simulink model "Sistema_Teste_Hugo_1"  (R2019a)
settings: Solver=ode23t  StartTime=0.0  StopTime=86400  MaxStep=6  RelTol=1e-3  EnableMultiTasking=on
InitFcn:
  | Dados_do_Sistema
undefined symbols (not defined in the file or in its folder): D1, Dados, Delta
libraries: powerlib x263, powerlib_meascontrol x79, dspsrcs4 x50
(part 3 of 5)

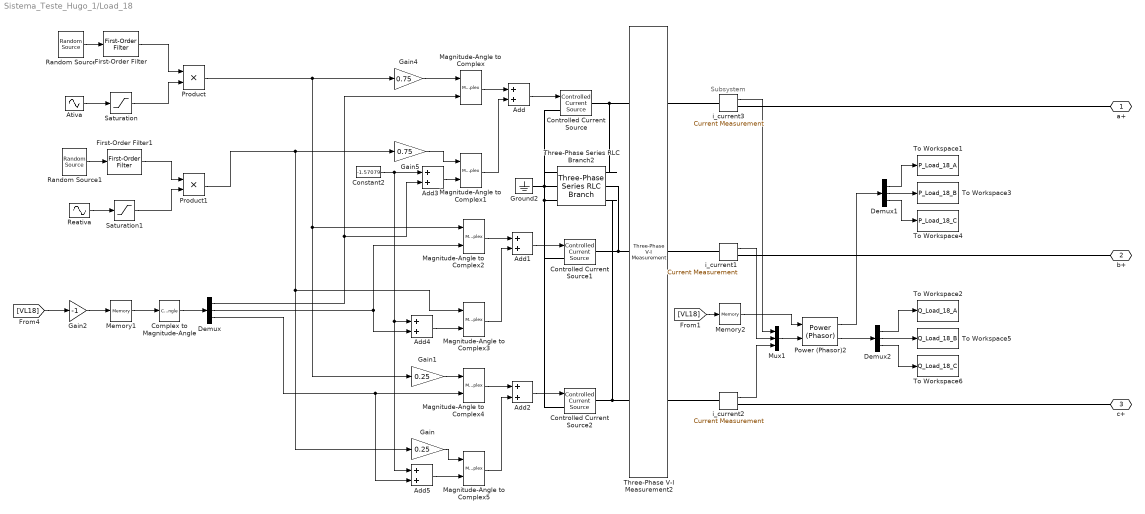
== system Sistema_Teste_Hugo_1/Load_18 ==
  note: Subsystem
  Add{,1..5} (6 alike) : Sum
  Ativa : Sin  Amplitude=21  Frequency=6.9e-5  Phase=-3.14  SampleTime=0
  Complex to Magnitude-Angle : ComplexToMagnitudeAngle  Output=Angle
  Constant2 : Constant  Value=-1.57079
  Controlled Current Source : powerlib/Electrical Sources/Controlled Current Source  Initialize=off  Source_Type=AC  Amplitude=0  Phase=0  Frequency=0  Measurements=None
      settings: SourceProductName=Simscape Electrical
  Controlled Current Source1 : powerlib/Electrical Sources/Controlled Current Source  Initialize=off  Source_Type=AC  Amplitude=0  Phase=0  Frequency=0  Measurements=None
      settings: SourceProductName=Simscape Electrical
  Controlled Current Source2 : powerlib/Electrical Sources/Controlled Current Source  Initialize=off  Source_Type=AC  Amplitude=0  Phase=0  Frequency=0  Measurements=None
      settings: SourceProductName=Simscape Electrical
  Demux : Demux  Outputs=3
  Demux1 : Demux  Outputs=3
  Demux2 : Demux  Outputs=3
  First-Order Filter : powerlib_meascontrol/Filters/First-Order Filter  FilterType=Lowpass  Tc=200  Ts=0  Initialize=on  Vac_Init=[0, 0, 60]  Vdc_Init=1  PlotResponse=off  FreqRange="[0,  200,  1]"
      settings: SourceProductName=Simscape Electrical
  First-Order Filter1 : powerlib_meascontrol/Filters/First-Order Filter  FilterType=Lowpass  Tc=400  Ts=0  Initialize=on  Vac_Init=[0, 0, 60]  Vdc_Init=1  PlotResponse=off  FreqRange="[0,  200,  1]"
      settings: SourceProductName=Simscape Electrical
  Gain : Gain  Gain=0.25
  Gain1 : Gain  Gain=0.25
  Gain2 : Gain  Gain=-1
  Gain4 : Gain  Gain=0.75
  Gain5 : Gain  Gain=0.75
  Ground2 : powerlib/Elements/Ground  LConnTagsString=a
      settings: SourceProductName=Simscape Electrical
  Magnitude-Angle to Complex{,1..5} (6 alike) : MagnitudeAngleToComplex
  Memory1 : Memory
  Memory2 : Memory
  Mux1 : Mux  Inputs=3
  Power (Phasor)2 : powerlib_meascontrol/Measurements/Power (Phasor)
      settings: SourceProductName=Simscape Electrical  SourceProductBaseCode=PS
  Product : Product
  Product1 : Product
  Random Source : dspsrcs4/Random Source  SrcType=Uniform  NormMethod=Ziggurat  CltLength=12  MinVal=0.4  MaxVal=1  MeanVal=0  VarVal=1  RepMode=Repeatable  rawSeed=1  IsInherit=off  SampMode=Discrete  SampTime=200  SampFrame=1  DataType=Single  OutComplex=Real  OutputFrames=on
  Random Source1 : dspsrcs4/Random Source  SrcType=Uniform  NormMethod=Ziggurat  CltLength=12  MinVal=0.75  MaxVal=1.1  MeanVal=0  VarVal=1  RepMode=Repeatable  rawSeed=1  IsInherit=off  SampMode=Discrete  SampTime=400  SampFrame=1  DataType=Single  OutComplex=Real  OutputFrames=on
  Reativa : Sin  Amplitude=9  Frequency=6.9e-5  Phase=-3.14  SampleTime=0
  Saturation : Saturate  UpperLimit=36  LowerLimit=10
  Saturation1 : Saturate  UpperLimit=10  LowerLimit=4
  Three-Phase Series RLC Branch2 : powerlib/Elements/Three-Phase Series RLC Branch  LConnTagsString=A|B|C  RConnTagsString=A|B|C  BranchType=RC  Resistance=0.0001  Inductance=5.46e-6  Capacitance=1e-9  Measurements=None
      settings: SourceProductName=Simscape Electrical
  Three-Phase V-I Measurement2 : powerlib/Measurements/Three-Phase V-I Measurement  VoltageMeasurement=phase-to-ground  SetLabelV=on  LabelV=VL18  Vpu=off  VpuLL=off  CurrentMeasurement=no  SetLabelI=on  LabelI=IL18  Ipu=off  Pbase=100e6  Vbase=500e3  OutputType=Complex  PhasorSimulation=on  PSBequivalent=0
      settings: SourceProductName=Simscape Electrical
  To Workspace1 : ToWorkspace  VariableName=P_Load_18_A  SampleTime=-1
  To Workspace2 : ToWorkspace  VariableName=Q_Load_18_A  SampleTime=-1
  To Workspace3 : ToWorkspace  VariableName=P_Load_18_B  SampleTime=-1
  To Workspace4 : ToWorkspace  VariableName=P_Load_18_C  SampleTime=-1
  To Workspace5 : ToWorkspace  VariableName=Q_Load_18_B  SampleTime=-1
  To Workspace6 : ToWorkspace  VariableName=Q_Load_18_C  SampleTime=-1
  i_current1 : powerlib/Measurements/Current Measurement  PhasorSimulation=on  OutputType=Complex  PSBequivalent=0
      settings: SourceProductName=Simscape Electrical
  i_current2 : powerlib/Measurements/Current Measurement  PhasorSimulation=on  OutputType=Complex  PSBequivalent=0
      settings: SourceProductName=Simscape Electrical
  i_current3 : powerlib/Measurements/Current Measurement  PhasorSimulation=on  OutputType=Complex  PSBequivalent=0
      settings: SourceProductName=Simscape Electrical
  a+ : PMIOPort  Side=Right
  b+ : PMIOPort  Port=2  Side=Right
  c+ : PMIOPort  Port=3  Side=Right
  wires:
  Ativa/1 -> Saturation/1
  Saturation/1 -> Product/2
  Random Source/1 -> First-Order Filter/1
  First-Order Filter/1 -> Product/1
  Reativa/1 -> Saturation1/1
  First-Order Filter1/1 -> Product1/1
  Random Source1/1 -> First-Order Filter1/1
  Saturation1/1 -> Product1/2
  Add/1 -> Controlled Current Source/1
  Magnitude-Angle to Complex/1 -> Add/1
  Magnitude-Angle to Complex1/1 -> Add/2
  Add1/1 -> Controlled Current Source1/1
  Magnitude-Angle to Complex2/1 -> Add1/1
  Magnitude-Angle to Complex3/1 -> Add1/2
  Add2/1 -> Controlled Current Source2/1
  Magnitude-Angle to Complex4/1 -> Add2/1
  Magnitude-Angle to Complex5/1 -> Add2/2
  Complex to Magnitude-Angle/1 -> Demux/1
  Demux/1 -> Magnitude-Angle to Complex/2, Add3/2
  Constant2/1 -> Add5/1, Add4/1, Add3/1
  Add3/1 -> Magnitude-Angle to Complex1/2
  Demux/2 -> Add4/2, Magnitude-Angle to Complex2/2
  Add4/1 -> Magnitude-Angle to Complex3/2
  Demux/3 -> Magnitude-Angle to Complex4/2, Add5/2
  Add5/1 -> Magnitude-Angle to Complex5/2
  [VL18] -> Gain2/1
  Memory1/1 -> Complex to Magnitude-Angle/1
  Product/1 -> Gain4/1, Magnitude-Angle to Complex2/1, Gain1/1
  Product1/1 -> Magnitude-Angle to Complex3/1, Gain/1, Gain5/1
  Gain1/1 -> Magnitude-Angle to Complex4/1
  Gain/1 -> Magnitude-Angle to Complex5/1
  Gain4/1 -> Magnitude-Angle to Complex/1
  Gain5/1 -> Magnitude-Angle to Complex1/1
  Gain2/1 -> Memory1/1
  Demux1/1 -> To Workspace1/1
  i_current3/1 -> Mux1/1
  Demux1/3 -> To Workspace4/1
  Demux2/2 -> To Workspace5/1
  Demux2/3 -> To Workspace6/1
  Memory2/1 -> Power (Phasor)2/1
  Demux1/2 -> To Workspace3/1
  i_current2/1 -> Mux1/3
  i_current1/1 -> Mux1/2
  Demux2/1 -> To Workspace2/1
  Mux1/1 -> Power (Phasor)2/2
  Power (Phasor)2/2 -> Demux2/1
  [VL18] -> Memory2/1
  Power (Phasor)2/1 -> Demux1/1
  connections:
  Controlled Current Source/RConn1 -- Three-Phase Series RLC Branch2/LConn1 -- Three-Phase V-I Measurement2/RConn1
  Controlled Current Source1/RConn1 -- Three-Phase Series RLC Branch2/LConn2 -- Three-Phase V-I Measurement2/RConn2
  Controlled Current Source2/RConn1 -- Three-Phase Series RLC Branch2/LConn3 -- Three-Phase V-I Measurement2/RConn3
  Ground2/LConn1 -- Controlled Current Source1/LConn1 -- Controlled Current Source2/LConn1 -- Three-Phase Series RLC Branch2/RConn3 -- Three-Phase Series RLC Branch2/RConn1 -- Controlled Current Source/LConn1 -- Three-Phase Series RLC Branch2/RConn2
  Three-Phase V-I Measurement2/LConn2 -- i_current1/LConn1
  a+/RConn1 -- i_current3/RConn1
  c+/RConn1 -- i_current2/RConn1
  b+/RConn1 -- i_current1/RConn1
  Three-Phase V-I Measurement2/LConn1 -- i_current3/LConn1
  Three-Phase V-I Measurement2/LConn3 -- i_current2/LConn1

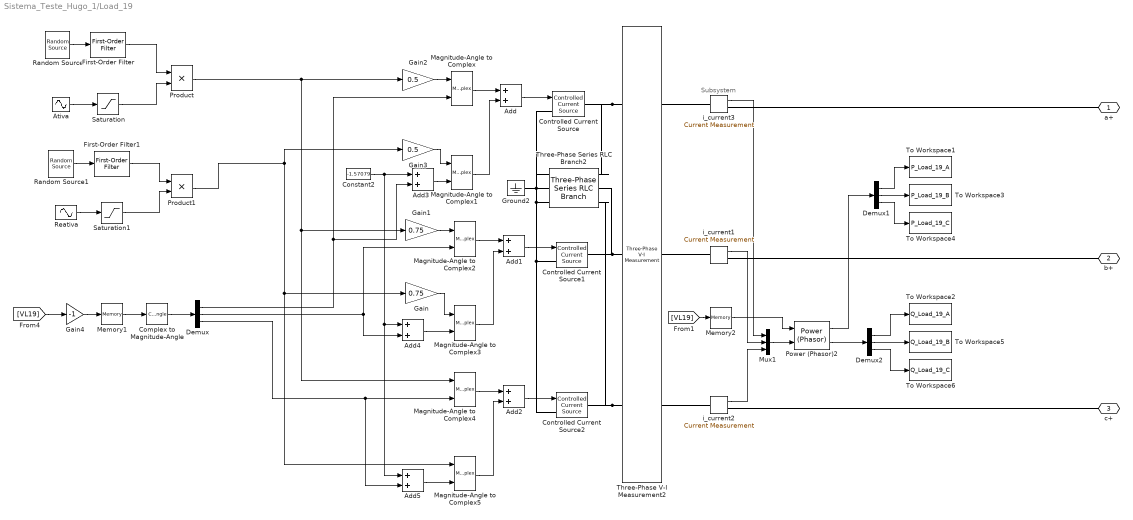
== system Sistema_Teste_Hugo_1/Load_19 ==
  note: Subsystem
  Add{,1..5} (6 alike) : Sum
  Ativa : Sin  Amplitude=22  Frequency=6.9e-5  Phase=-3.14  SampleTime=0
  Complex to Magnitude-Angle : ComplexToMagnitudeAngle  Output=Angle
  Constant2 : Constant  Value=-1.57079
  Controlled Current Source : powerlib/Electrical Sources/Controlled Current Source  Initialize=off  Source_Type=AC  Amplitude=0  Phase=0  Frequency=0  Measurements=None
      settings: SourceProductName=Simscape Electrical
  Controlled Current Source1 : powerlib/Electrical Sources/Controlled Current Source  Initialize=off  Source_Type=AC  Amplitude=0  Phase=0  Frequency=0  Measurements=None
      settings: SourceProductName=Simscape Electrical
  Controlled Current Source2 : powerlib/Electrical Sources/Controlled Current Source  Initialize=off  Source_Type=AC  Amplitude=0  Phase=0  Frequency=0  Measurements=None
      settings: SourceProductName=Simscape Electrical
  Demux : Demux  Outputs=3
  Demux1 : Demux  Outputs=3
  Demux2 : Demux  Outputs=3
  First-Order Filter : powerlib_meascontrol/Filters/First-Order Filter  FilterType=Lowpass  Tc=200  Ts=0  Initialize=on  Vac_Init=[0, 0, 60]  Vdc_Init=1  PlotResponse=off  FreqRange="[0,  200,  1]"
      settings: SourceProductName=Simscape Electrical
  First-Order Filter1 : powerlib_meascontrol/Filters/First-Order Filter  FilterType=Lowpass  Tc=400  Ts=0  Initialize=on  Vac_Init=[0, 0, 60]  Vdc_Init=1  PlotResponse=off  FreqRange="[0,  200,  1]"
      settings: SourceProductName=Simscape Electrical
  Gain : Gain  Gain=0.75
  Gain1 : Gain  Gain=0.75
  Gain2 : Gain  Gain=0.5
  Gain3 : Gain  Gain=0.5
  Gain4 : Gain  Gain=-1
  Ground2 : powerlib/Elements/Ground  LConnTagsString=a
      settings: SourceProductName=Simscape Electrical
  Magnitude-Angle to Complex{,1..5} (6 alike) : MagnitudeAngleToComplex
  Memory1 : Memory
  Memory2 : Memory
  Mux1 : Mux  Inputs=3
  Power (Phasor)2 : powerlib_meascontrol/Measurements/Power (Phasor)
      settings: SourceProductName=Simscape Electrical  SourceProductBaseCode=PS
  Product : Product
  Product1 : Product
  Random Source : dspsrcs4/Random Source  SrcType=Uniform  NormMethod=Ziggurat  CltLength=12  MinVal=0.6  MaxVal=1  MeanVal=0  VarVal=1  RepMode=Repeatable  rawSeed=1  IsInherit=off  SampMode=Discrete  SampTime=200  SampFrame=1  DataType=Single  OutComplex=Real  OutputFrames=on
  Random Source1 : dspsrcs4/Random Source  SrcType=Uniform  NormMethod=Ziggurat  CltLength=12  MinVal=0.8  MaxVal=1  MeanVal=0  VarVal=1  RepMode=Repeatable  rawSeed=1  IsInherit=off  SampMode=Discrete  SampTime=400  SampFrame=1  DataType=Single  OutComplex=Real  OutputFrames=on
  Reativa : Sin  Amplitude=8  Frequency=6.9e-5  Phase=-3.14  SampleTime=0
  Saturation : Saturate  UpperLimit=24  LowerLimit=11
  Saturation1 : Saturate  UpperLimit=9  LowerLimit=7
  Three-Phase Series RLC Branch2 : powerlib/Elements/Three-Phase Series RLC Branch  LConnTagsString=A|B|C  RConnTagsString=A|B|C  BranchType=RC  Resistance=0.0001  Inductance=5.46e-6  Capacitance=1e-9  Measurements=None
      settings: SourceProductName=Simscape Electrical
  Three-Phase V-I Measurement2 : powerlib/Measurements/Three-Phase V-I Measurement  VoltageMeasurement=phase-to-ground  SetLabelV=on  LabelV=VL19  Vpu=off  VpuLL=off  CurrentMeasurement=no  SetLabelI=on  LabelI=IL19  Ipu=off  Pbase=100e6  Vbase=500e3  OutputType=Complex  PhasorSimulation=on  PSBequivalent=0
      settings: SourceProductName=Simscape Electrical
  To Workspace1 : ToWorkspace  VariableName=P_Load_19_A  SampleTime=-1
  To Workspace2 : ToWorkspace  VariableName=Q_Load_19_A  SampleTime=-1
  To Workspace3 : ToWorkspace  VariableName=P_Load_19_B  SampleTime=-1
  To Workspace4 : ToWorkspace  VariableName=P_Load_19_C  SampleTime=-1
  To Workspace5 : ToWorkspace  VariableName=Q_Load_19_B  SampleTime=-1
  To Workspace6 : ToWorkspace  VariableName=Q_Load_19_C  SampleTime=-1
  i_current1 : powerlib/Measurements/Current Measurement  PhasorSimulation=on  OutputType=Complex  PSBequivalent=0
      settings: SourceProductName=Simscape Electrical
  i_current2 : powerlib/Measurements/Current Measurement  PhasorSimulation=on  OutputType=Complex  PSBequivalent=0
      settings: SourceProductName=Simscape Electrical
  i_current3 : powerlib/Measurements/Current Measurement  PhasorSimulation=on  OutputType=Complex  PSBequivalent=0
      settings: SourceProductName=Simscape Electrical
  a+ : PMIOPort  Side=Right
  b+ : PMIOPort  Port=2  Side=Right
  c+ : PMIOPort  Port=3  Side=Right
  wires:
  Ativa/1 -> Saturation/1
  Saturation/1 -> Product/2
  Random Source/1 -> First-Order Filter/1
  First-Order Filter/1 -> Product/1
  Reativa/1 -> Saturation1/1
  First-Order Filter1/1 -> Product1/1
  Random Source1/1 -> First-Order Filter1/1
  Saturation1/1 -> Product1/2
  Add/1 -> Controlled Current Source/1
  Magnitude-Angle to Complex/1 -> Add/1
  Magnitude-Angle to Complex1/1 -> Add/2
  Add1/1 -> Controlled Current Source1/1
  Magnitude-Angle to Complex2/1 -> Add1/1
  Magnitude-Angle to Complex3/1 -> Add1/2
  Add2/1 -> Controlled Current Source2/1
  Magnitude-Angle to Complex4/1 -> Add2/1
  Magnitude-Angle to Complex5/1 -> Add2/2
  Complex to Magnitude-Angle/1 -> Demux/1
  Demux/1 -> Magnitude-Angle to Complex/2, Add3/2
  Constant2/1 -> Add5/1, Add4/1, Add3/1
  Add3/1 -> Magnitude-Angle to Complex1/2
  Demux/2 -> Add4/2, Magnitude-Angle to Complex2/2
  Add4/1 -> Magnitude-Angle to Complex3/2
  Demux/3 -> Magnitude-Angle to Complex4/2, Add5/2
  Add5/1 -> Magnitude-Angle to Complex5/2
  [VL19] -> Gain4/1
  Memory1/1 -> Complex to Magnitude-Angle/1
  Gain1/1 -> Magnitude-Angle to Complex2/1
  Gain/1 -> Magnitude-Angle to Complex3/1
  Product/1 -> Gain2/1, Magnitude-Angle to Complex4/1, Gain1/1
  Product1/1 -> Gain3/1, Magnitude-Angle to Complex5/1, Gain/1
  Gain4/1 -> Memory1/1
  Gain2/1 -> Magnitude-Angle to Complex/1
  Gain3/1 -> Magnitude-Angle to Complex1/1
  Power (Phasor)2/2 -> Demux2/1
  Demux2/1 -> To Workspace2/1
  Power (Phasor)2/1 -> Demux1/1
  i_current3/1 -> Mux1/1
  i_current1/1 -> Mux1/2
  Demux2/3 -> To Workspace6/1
  Demux1/3 -> To Workspace4/1
  Memory2/1 -> Power (Phasor)2/1
  Demux2/2 -> To Workspace5/1
  i_current2/1 -> Mux1/3
  [VL19] -> Memory2/1
  Demux1/1 -> To Workspace1/1
  Demux1/2 -> To Workspace3/1
  Mux1/1 -> Power (Phasor)2/2
  connections:
  Three-Phase V-I Measurement2/RConn1 -- Controlled Current Source/RConn1 -- Three-Phase Series RLC Branch2/LConn1
  Three-Phase V-I Measurement2/RConn2 -- Controlled Current Source1/RConn1 -- Three-Phase Series RLC Branch2/LConn2
  Three-Phase V-I Measurement2/RConn3 -- Controlled Current Source2/RConn1 -- Three-Phase Series RLC Branch2/LConn3
  Controlled Current Source1/LConn1 -- Three-Phase Series RLC Branch2/RConn3 -- Three-Phase Series RLC Branch2/RConn1 -- Controlled Current Source/LConn1 -- Three-Phase Series RLC Branch2/RConn2 -- Ground2/LConn1 -- Controlled Current Source2/LConn1
  b+/RConn1 -- i_current1/RConn1
  c+/RConn1 -- i_current2/RConn1
  Three-Phase V-I Measurement2/LConn2 -- i_current1/LConn1
  a+/RConn1 -- i_current3/RConn1
  Three-Phase V-I Measurement2/LConn3 -- i_current2/LConn1
  Three-Phase V-I Measurement2/LConn1 -- i_current3/LConn1

== system Sistema_Teste_Hugo_1/Load_21 ==
  note: Subsystem
  Add{,1..5} (6 alike) : Sum
  Ativa : Sin  Amplitude=16  Frequency=6.9e-5  Phase=-3.14  SampleTime=0
  Complex to Magnitude-Angle : ComplexToMagnitudeAngle  Output=Angle
  Constant2 : Constant  Value=-1.57079
  Controlled Current Source : powerlib/Electrical Sources/Controlled Current Source  Initialize=off  Source_Type=AC  Amplitude=0  Phase=0  Frequency=0  Measurements=None
      settings: SourceProductName=Simscape Electrical
  Controlled Current Source1 : powerlib/Electrical Sources/Controlled Current Source  Initialize=off  Source_Type=AC  Amplitude=0  Phase=0  Frequency=0  Measurements=None
      settings: SourceProductName=Simscape Electrical
  Controlled Current Source2 : powerlib/Electrical Sources/Controlled Current Source  Initialize=off  Source_Type=AC  Amplitude=0  Phase=0  Frequency=0  Measurements=None
      settings: SourceProductName=Simscape Electrical
  Demux : Demux  Outputs=3
  Demux1 : Demux  Outputs=3
  Demux2 : Demux  Outputs=3
  First-Order Filter : powerlib_meascontrol/Filters/First-Order Filter  FilterType=Lowpass  Tc=200  Ts=0  Initialize=on  Vac_Init=[0, 0, 60]  Vdc_Init=1  PlotResponse=off  FreqRange="[0,  200,  1]"
      settings: SourceProductName=Simscape Electrical
  First-Order Filter1 : powerlib_meascontrol/Filters/First-Order Filter  FilterType=Lowpass  Tc=400  Ts=0  Initialize=on  Vac_Init=[0, 0, 60]  Vdc_Init=1  PlotResponse=off  FreqRange="[0,  200,  1]"
      settings: SourceProductName=Simscape Electrical
  Gain : Gain  Gain=0.25
  Gain1 : Gain  Gain=0.25
  Gain2 : Gain  Gain=0
  Gain3 : Gain  Gain=0
  Gain4 : Gain  Gain=-1
  Ground2 : powerlib/Elements/Ground  LConnTagsString=a
      settings: SourceProductName=Simscape Electrical
  Magnitude-Angle to Complex{,1..5} (6 alike) : MagnitudeAngleToComplex
  Memory1 : Memory
  Memory2 : Memory
  Mux1 : Mux  Inputs=3
  Power (Phasor)2 : powerlib_meascontrol/Measurements/Power (Phasor)
      settings: SourceProductName=Simscape Electrical  SourceProductBaseCode=PS
  Product : Product
  Product1 : Product
  Random Source : dspsrcs4/Random Source  SrcType=Uniform  NormMethod=Ziggurat  CltLength=12  MinVal=0.75  MaxVal=1  MeanVal=0  VarVal=1  RepMode=Repeatable  rawSeed=1  IsInherit=off  SampMode=Discrete  SampTime=200  SampFrame=1  DataType=Single  OutComplex=Real  OutputFrames=on
  Random Source1 : dspsrcs4/Random Source  SrcType=Uniform  NormMethod=Ziggurat  CltLength=12  MinVal=0.8  MaxVal=1  MeanVal=0  VarVal=1  RepMode=Repeatable  rawSeed=1  IsInherit=off  SampMode=Discrete  SampTime=400  SampFrame=1  DataType=Single  OutComplex=Real  OutputFrames=on
  Reativa : Sin  Amplitude=9  Frequency=6.9e-5  Phase=-3.14  SampleTime=0
  Saturation : Saturate  UpperLimit=24  LowerLimit=14
  Saturation1 : Saturate  UpperLimit=12  LowerLimit=8
  Three-Phase Series RLC Branch2 : powerlib/Elements/Three-Phase Series RLC Branch  LConnTagsString=A|B|C  RConnTagsString=A|B|C  BranchType=RC  Resistance=0.0001  Inductance=5.46e-6  Capacitance=1e-9  Measurements=None
      settings: SourceProductName=Simscape Electrical
  Three-Phase V-I Measurement2 : powerlib/Measurements/Three-Phase V-I Measurement  VoltageMeasurement=phase-to-ground  SetLabelV=on  LabelV=VL21  Vpu=off  VpuLL=off  CurrentMeasurement=no  SetLabelI=on  LabelI=IL21  Ipu=off  Pbase=100e6  Vbase=500e3  OutputType=Complex  PhasorSimulation=on  PSBequivalent=0
      settings: SourceProductName=Simscape Electrical
  To Workspace1 : ToWorkspace  VariableName=P_Load_21_A  SampleTime=-1
  To Workspace2 : ToWorkspace  VariableName=Q_Load_21_A  SampleTime=-1
  To Workspace3 : ToWorkspace  VariableName=P_Load_21_B  SampleTime=-1
  To Workspace4 : ToWorkspace  VariableName=P_Load_21_C  SampleTime=-1
  To Workspace5 : ToWorkspace  VariableName=Q_Load_21_B  SampleTime=-1
  To Workspace6 : ToWorkspace  VariableName=Q_Load_21_C  SampleTime=-1
  i_current1 : powerlib/Measurements/Current Measurement  PhasorSimulation=on  OutputType=Complex  PSBequivalent=0
      settings: SourceProductName=Simscape Electrical
  i_current2 : powerlib/Measurements/Current Measurement  PhasorSimulation=on  OutputType=Complex  PSBequivalent=0
      settings: SourceProductName=Simscape Electrical
  i_current3 : powerlib/Measurements/Current Measurement  PhasorSimulation=on  OutputType=Complex  PSBequivalent=0
      settings: SourceProductName=Simscape Electrical
  a+ : PMIOPort  Side=Right
  b+ : PMIOPort  Port=2  Side=Right
  c+ : PMIOPort  Port=3  Side=Right
  wires:
  Ativa/1 -> Saturation/1
  Saturation/1 -> Product/2
  Random Source/1 -> First-Order Filter/1
  First-Order Filter/1 -> Product/1
  Reativa/1 -> Saturation1/1
  First-Order Filter1/1 -> Product1/1
  Random Source1/1 -> First-Order Filter1/1
  Saturation1/1 -> Product1/2
  Add/1 -> Controlled Current Source/1
  Magnitude-Angle to Complex/1 -> Add/1
  Magnitude-Angle to Complex1/1 -> Add/2
  Add1/1 -> Controlled Current Source1/1
  Magnitude-Angle to Complex2/1 -> Add1/1
  Magnitude-Angle to Complex3/1 -> Add1/2
  Add2/1 -> Controlled Current Source2/1
  Magnitude-Angle to Complex4/1 -> Add2/1
  Magnitude-Angle to Complex5/1 -> Add2/2
  Complex to Magnitude-Angle/1 -> Demux/1
  Demux/1 -> Magnitude-Angle to Complex/2, Add3/2
  Constant2/1 -> Add5/1, Add4/1, Add3/1
  Add3/1 -> Magnitude-Angle to Complex1/2
  Demux/2 -> Add4/2, Magnitude-Angle to Complex2/2
  Add4/1 -> Magnitude-Angle to Complex3/2
  Demux/3 -> Magnitude-Angle to Complex4/2, Add5/2
  Add5/1 -> Magnitude-Angle to Complex5/2
  [VL21] -> Gain4/1
  Memory1/1 -> Complex to Magnitude-Angle/1
  Product/1 -> Gain2/1, Magnitude-Angle to Complex2/1, Gain1/1
  Product1/1 -> Gain3/1, Magnitude-Angle to Complex3/1, Gain/1
  Gain4/1 -> Memory1/1
  Gain2/1 -> Magnitude-Angle to Complex/1
  Gain3/1 -> Magnitude-Angle to Complex1/1
  Gain/1 -> Magnitude-Angle to Complex5/1
  Gain1/1 -> Magnitude-Angle to Complex4/1
  Demux2/2 -> To Workspace5/1
  [VL21] -> Memory2/1
  Memory2/1 -> Power (Phasor)2/1
  Demux1/1 -> To Workspace1/1
  i_current2/1 -> Mux1/3
  i_current3/1 -> Mux1/1
  Power (Phasor)2/1 -> Demux1/1
  Demux1/2 -> To Workspace3/1
  i_current1/1 -> Mux1/2
  Demux2/1 -> To Workspace2/1
  Power (Phasor)2/2 -> Demux2/1
  Demux2/3 -> To Workspace6/1
  Mux1/1 -> Power (Phasor)2/2
  Demux1/3 -> To Workspace4/1
  connections:
  Three-Phase V-I Measurement2/RConn1 -- Controlled Current Source/RConn1 -- Three-Phase Series RLC Branch2/LConn1
  Three-Phase V-I Measurement2/RConn2 -- Controlled Current Source1/RConn1 -- Three-Phase Series RLC Branch2/LConn2
  Three-Phase V-I Measurement2/RConn3 -- Controlled Current Source2/RConn1 -- Three-Phase Series RLC Branch2/LConn3
  Controlled Current Source1/LConn1 -- Three-Phase Series RLC Branch2/RConn3 -- Three-Phase Series RLC Branch2/RConn1 -- Controlled Current Source/LConn1 -- Three-Phase Series RLC Branch2/RConn2 -- Ground2/LConn1 -- Controlled Current Source2/LConn1
  a+/RConn1 -- i_current3/RConn1
  b+/RConn1 -- i_current1/RConn1
  Three-Phase V-I Measurement2/LConn2 -- i_current1/LConn1
  Three-Phase V-I Measurement2/LConn3 -- i_current2/LConn1
  c+/RConn1 -- i_current2/RConn1
  Three-Phase V-I Measurement2/LConn1 -- i_current3/LConn1

== system Sistema_Teste_Hugo_1/Load_23 ==
  note: Subsystem
  Add{,1..5} (6 alike) : Sum
  Ativa : Sin  Amplitude=22  Frequency=6.9e-5  Phase=-3.14  SampleTime=0
  Complex to Magnitude-Angle : ComplexToMagnitudeAngle  Output=Angle
  Constant2 : Constant  Value=-1.57079
  Controlled Current Source : powerlib/Electrical Sources/Controlled Current Source  Initialize=off  Source_Type=AC  Amplitude=0  Phase=0  Frequency=0  Measurements=None
      settings: SourceProductName=Simscape Electrical
  Controlled Current Source1 : powerlib/Electrical Sources/Controlled Current Source  Initialize=off  Source_Type=AC  Amplitude=0  Phase=0  Frequency=0  Measurements=None
      settings: SourceProductName=Simscape Electrical
  Controlled Current Source2 : powerlib/Electrical Sources/Controlled Current Source  Initialize=off  Source_Type=AC  Amplitude=0  Phase=0  Frequency=0  Measurements=None
      settings: SourceProductName=Simscape Electrical
  Demux : Demux  Outputs=3
  Demux1 : Demux  Outputs=3
  Demux2 : Demux  Outputs=3
  First-Order Filter : powerlib_meascontrol/Filters/First-Order Filter  FilterType=Lowpass  Tc=200  Ts=0  Initialize=on  Vac_Init=[0, 0, 60]  Vdc_Init=1  PlotResponse=off  FreqRange="[0,  200,  1]"
      settings: SourceProductName=Simscape Electrical
  First-Order Filter1 : powerlib_meascontrol/Filters/First-Order Filter  FilterType=Lowpass  Tc=400  Ts=0  Initialize=on  Vac_Init=[0, 0, 60]  Vdc_Init=1  PlotResponse=off  FreqRange="[0,  200,  1]"
      settings: SourceProductName=Simscape Electrical
  Gain : Gain  Gain=1.25
  Gain1 : Gain  Gain=1.25
  Gain2 : Gain  Gain=2
  Gain3 : Gain  Gain=2
  Gain4 : Gain  Gain=-1
  Ground2 : powerlib/Elements/Ground  LConnTagsString=a
      settings: SourceProductName=Simscape Electrical
  Magnitude-Angle to Complex{,1..5} (6 alike) : MagnitudeAngleToComplex
  Memory1 : Memory
  Memory2 : Memory
  Mux1 : Mux  Inputs=3
  Power (Phasor)2 : powerlib_meascontrol/Measurements/Power (Phasor)
      settings: SourceProductName=Simscape Electrical  SourceProductBaseCode=PS
  Product : Product
  Product1 : Product
  Random Source : dspsrcs4/Random Source  SrcType=Uniform  NormMethod=Ziggurat  CltLength=12  MinVal=0.65  MaxVal=1  MeanVal=0  VarVal=1  RepMode=Repeatable  rawSeed=1  IsInherit=off  SampMode=Discrete  SampTime=200  SampFrame=1  DataType=Single  OutComplex=Real  OutputFrames=on
  Random Source1 : dspsrcs4/Random Source  SrcType=Uniform  NormMethod=Ziggurat  CltLength=12  MinVal=0.7  MaxVal=1  MeanVal=0  VarVal=1  RepMode=Repeatable  rawSeed=1  IsInherit=off  SampMode=Discrete  SampTime=400  SampFrame=1  DataType=Single  OutComplex=Real  OutputFrames=on
  Reativa : Sin  Amplitude=11  Frequency=6.9e-5  Phase=-3.14  SampleTime=0
  Saturation : Saturate  UpperLimit=24  LowerLimit=14
  Saturation1 : Saturate  UpperLimit=15  LowerLimit=7
  Three-Phase Series RLC Branch2 : powerlib/Elements/Three-Phase Series RLC Branch  LConnTagsString=A|B|C  RConnTagsString=A|B|C  BranchType=RC  Resistance=0.0001  Inductance=5.46e-6  Capacitance=1e-9  Measurements=None
      settings: SourceProductName=Simscape Electrical
  Three-Phase V-I Measurement2 : powerlib/Measurements/Three-Phase V-I Measurement  VoltageMeasurement=phase-to-ground  SetLabelV=on  LabelV=VL23  Vpu=off  VpuLL=off  CurrentMeasurement=no  SetLabelI=on  LabelI=IL23  Ipu=off  Pbase=100e6  Vbase=500e3  OutputType=Complex  PhasorSimulation=on  PSBequivalent=0
      settings: SourceProductName=Simscape Electrical
  To Workspace1 : ToWorkspace  VariableName=P_Load_23_A  SampleTime=-1
  To Workspace2 : ToWorkspace  VariableName=Q_Load_23_A  SampleTime=-1
  To Workspace3 : ToWorkspace  VariableName=P_Load_23_B  SampleTime=-1
  To Workspace4 : ToWorkspace  VariableName=P_Load_23_C  SampleTime=-1
  To Workspace5 : ToWorkspace  VariableName=Q_Load_23_B  SampleTime=-1
  To Workspace6 : ToWorkspace  VariableName=Q_Load_23_C  SampleTime=-1
  i_current1 : powerlib/Measurements/Current Measurement  PhasorSimulation=on  OutputType=Complex  PSBequivalent=0
      settings: SourceProductName=Simscape Electrical
  i_current2 : powerlib/Measurements/Current Measurement  PhasorSimulation=on  OutputType=Complex  PSBequivalent=0
      settings: SourceProductName=Simscape Electrical
  i_current3 : powerlib/Measurements/Current Measurement  PhasorSimulation=on  OutputType=Complex  PSBequivalent=0
      settings: SourceProductName=Simscape Electrical
  a+ : PMIOPort  Side=Right
  b+ : PMIOPort  Port=2  Side=Right
  c+ : PMIOPort  Port=3  Side=Right
  wires:
  Ativa/1 -> Saturation/1
  Saturation/1 -> Product/2
  Random Source/1 -> First-Order Filter/1
  First-Order Filter/1 -> Product/1
  Reativa/1 -> Saturation1/1
  First-Order Filter1/1 -> Product1/1
  Random Source1/1 -> First-Order Filter1/1
  Saturation1/1 -> Product1/2
  Add/1 -> Controlled Current Source/1
  Magnitude-Angle to Complex/1 -> Add/1
  Magnitude-Angle to Complex1/1 -> Add/2
  Add1/1 -> Controlled Current Source1/1
  Magnitude-Angle to Complex2/1 -> Add1/1
  Magnitude-Angle to Complex3/1 -> Add1/2
  Add2/1 -> Controlled Current Source2/1
  Magnitude-Angle to Complex4/1 -> Add2/1
  Magnitude-Angle to Complex5/1 -> Add2/2
  Complex to Magnitude-Angle/1 -> Demux/1
  Demux/1 -> Magnitude-Angle to Complex/2, Add3/2
  Constant2/1 -> Add5/1, Add4/1, Add3/1
  Add3/1 -> Magnitude-Angle to Complex1/2
  Demux/2 -> Add4/2, Magnitude-Angle to Complex2/2
  Add4/1 -> Magnitude-Angle to Complex3/2
  Demux/3 -> Magnitude-Angle to Complex4/2, Add5/2
  Add5/1 -> Magnitude-Angle to Complex5/2
  [VL23] -> Gain4/1
  Memory1/1 -> Complex to Magnitude-Angle/1
  Product/1 -> Gain2/1, Magnitude-Angle to Complex2/1, Gain1/1
  Product1/1 -> Gain3/1, Magnitude-Angle to Complex3/1, Gain/1
  Gain4/1 -> Memory1/1
  Gain2/1 -> Magnitude-Angle to Complex/1
  Gain3/1 -> Magnitude-Angle to Complex1/1
  Gain1/1 -> Magnitude-Angle to Complex4/1
  Gain/1 -> Magnitude-Angle to Complex5/1
  Demux2/3 -> To Workspace6/1
  Demux2/1 -> To Workspace2/1
  Mux1/1 -> Power (Phasor)2/2
  Power (Phasor)2/2 -> Demux2/1
  Demux1/3 -> To Workspace4/1
  i_current1/1 -> Mux1/2
  Power (Phasor)2/1 -> Demux1/1
  i_current3/1 -> Mux1/1
  Demux1/2 -> To Workspace3/1
  i_current2/1 -> Mux1/3
  Memory2/1 -> Power (Phasor)2/1
  Demux2/2 -> To Workspace5/1
  Demux1/1 -> To Workspace1/1
  [VL23] -> Memory2/1
  connections:
  Three-Phase V-I Measurement2/RConn1 -- Controlled Current Source/RConn1 -- Three-Phase Series RLC Branch2/LConn1
  Three-Phase V-I Measurement2/RConn2 -- Controlled Current Source1/RConn1 -- Three-Phase Series RLC Branch2/LConn2
  Three-Phase V-I Measurement2/RConn3 -- Controlled Current Source2/RConn1 -- Three-Phase Series RLC Branch2/LConn3
  Controlled Current Source1/LConn1 -- Three-Phase Series RLC Branch2/RConn3 -- Three-Phase Series RLC Branch2/RConn1 -- Controlled Current Source/LConn1 -- Three-Phase Series RLC Branch2/RConn2 -- Ground2/LConn1 -- Controlled Current Source2/LConn1
  Three-Phase V-I Measurement2/LConn1 -- i_current3/LConn1
  Three-Phase V-I Measurement2/LConn2 -- i_current1/LConn1
  b+/RConn1 -- i_current1/RConn1
  a+/RConn1 -- i_current3/RConn1
  c+/RConn1 -- i_current2/RConn1
  Three-Phase V-I Measurement2/LConn3 -- i_current2/LConn1

== system Sistema_Teste_Hugo_1/Load_25 ==
  note: Subsystem
  Add{,1..5} (6 alike) : Sum
  Ativa : Sin  Amplitude=10  Frequency=6.9e-5  Phase=-3.14  SampleTime=0
  Complex to Magnitude-Angle : ComplexToMagnitudeAngle  Output=Angle
  Constant2 : Constant  Value=-1.57079
  Controlled Current Source : powerlib/Electrical Sources/Controlled Current Source  Initialize=off  Source_Type=AC  Amplitude=0  Phase=0  Frequency=0  Measurements=None
      settings: SourceProductName=Simscape Electrical
  Controlled Current Source1 : powerlib/Electrical Sources/Controlled Current Source  Initialize=off  Source_Type=AC  Amplitude=0  Phase=0  Frequency=0  Measurements=None
      settings: SourceProductName=Simscape Electrical
  Controlled Current Source2 : powerlib/Electrical Sources/Controlled Current Source  Initialize=off  Source_Type=AC  Amplitude=0  Phase=0  Frequency=0  Measurements=None
      settings: SourceProductName=Simscape Electrical
  Demux : Demux  Outputs=3
  Demux1 : Demux  Outputs=3
  Demux2 : Demux  Outputs=3
  First-Order Filter : powerlib_meascontrol/Filters/First-Order Filter  FilterType=Lowpass  Tc=200  Ts=0  Initialize=on  Vac_Init=[0, 0, 60]  Vdc_Init=1  PlotResponse=off  FreqRange="[0,  200,  1]"
      settings: SourceProductName=Simscape Electrical
  First-Order Filter1 : powerlib_meascontrol/Filters/First-Order Filter  FilterType=Lowpass  Tc=400  Ts=0  Initialize=on  Vac_Init=[0, 0, 60]  Vdc_Init=1  PlotResponse=off  FreqRange="[0,  200,  1]"
      settings: SourceProductName=Simscape Electrical
  Gain2 : Gain  Gain=1.25
  Gain4 : Gain  Gain=-1
  Ground2 : powerlib/Elements/Ground  LConnTagsString=a
      settings: SourceProductName=Simscape Electrical
  Magnitude-Angle to Complex{,1..5} (6 alike) : MagnitudeAngleToComplex
  Memory1 : Memory
  Memory2 : Memory
  Mux1 : Mux  Inputs=3
  Power (Phasor)2 : powerlib_meascontrol/Measurements/Power (Phasor)
      settings: SourceProductName=Simscape Electrical  SourceProductBaseCode=PS
  Product : Product
  Product1 : Product
  Random Source : dspsrcs4/Random Source  SrcType=Uniform  NormMethod=Ziggurat  CltLength=12  MinVal=0.6  MaxVal=1  MeanVal=0  VarVal=1  RepMode=Repeatable  rawSeed=1  IsInherit=off  SampMode=Discrete  SampTime=200  SampFrame=1  DataType=Single  OutComplex=Real  OutputFrames=on
  Random Source1 : dspsrcs4/Random Source  SrcType=Uniform  NormMethod=Ziggurat  CltLength=12  MinVal=0.8  MaxVal=1.05  MeanVal=0  VarVal=1  RepMode=Repeatable  rawSeed=1  IsInherit=off  SampMode=Discrete  SampTime=400  SampFrame=1  DataType=Single  OutComplex=Real  OutputFrames=on
  Reativa : Sin  Amplitude=4  Frequency=6.9e-5  Phase=-3.14  SampleTime=0
  Saturation : Saturate  UpperLimit=36  LowerLimit=5
  Saturation1 : Saturate  UpperLimit=10  LowerLimit=3
  Three-Phase Series RLC Branch2 : powerlib/Elements/Three-Phase Series RLC Branch  LConnTagsString=A|B|C  RConnTagsString=A|B|C  BranchType=RC  Resistance=0.0001  Inductance=5.46e-6  Capacitance=1e-9  Measurements=None
      settings: SourceProductName=Simscape Electrical
  Three-Phase V-I Measurement2 : powerlib/Measurements/Three-Phase V-I Measurement  VoltageMeasurement=phase-to-ground  SetLabelV=on  LabelV=VL25  Vpu=off  VpuLL=off  CurrentMeasurement=no  SetLabelI=on  LabelI=IL25  Ipu=off  Pbase=100e6  Vbase=500e3  OutputType=Complex  PhasorSimulation=on  PSBequivalent=0
      settings: SourceProductName=Simscape Electrical
  To Workspace1 : ToWorkspace  VariableName=P_Load_25_A  SampleTime=-1
  To Workspace2 : ToWorkspace  VariableName=Q_Load_25_A  SampleTime=-1
  To Workspace3 : ToWorkspace  VariableName=P_Load_25_B  SampleTime=-1
  To Workspace4 : ToWorkspace  VariableName=P_Load_25_C  SampleTime=-1
  To Workspace5 : ToWorkspace  VariableName=Q_Load_25_B  SampleTime=-1
  To Workspace6 : ToWorkspace  VariableName=Q_Load_25_C  SampleTime=-1
  i_current1 : powerlib/Measurements/Current Measurement  PhasorSimulation=on  OutputType=Complex  PSBequivalent=0
      settings: SourceProductName=Simscape Electrical
  i_current2 : powerlib/Measurements/Current Measurement  PhasorSimulation=on  OutputType=Complex  PSBequivalent=0
      settings: SourceProductName=Simscape Electrical
  i_current3 : powerlib/Measurements/Current Measurement  PhasorSimulation=on  OutputType=Complex  PSBequivalent=0
      settings: SourceProductName=Simscape Electrical
  a+ : PMIOPort  Side=Right
  b+ : PMIOPort  Port=2  Side=Right
  c+ : PMIOPort  Port=3  Side=Right
  wires:
  Ativa/1 -> Saturation/1
  Saturation/1 -> Product/2
  Random Source/1 -> First-Order Filter/1
  First-Order Filter/1 -> Product/1
  Reativa/1 -> Saturation1/1
  First-Order Filter1/1 -> Product1/1
  Random Source1/1 -> First-Order Filter1/1
  Saturation1/1 -> Product1/2
  Add/1 -> Controlled Current Source/1
  Magnitude-Angle to Complex/1 -> Add/1
  Magnitude-Angle to Complex1/1 -> Add/2
  Add1/1 -> Controlled Current Source1/1
  Magnitude-Angle to Complex2/1 -> Add1/1
  Magnitude-Angle to Complex3/1 -> Add1/2
  Add2/1 -> Controlled Current Source2/1
  Magnitude-Angle to Complex4/1 -> Add2/1
  Magnitude-Angle to Complex5/1 -> Add2/2
  Complex to Magnitude-Angle/1 -> Demux/1
  Demux/1 -> Magnitude-Angle to Complex/2, Add3/2
  Constant2/1 -> Add5/1, Add4/1, Add3/1
  Add3/1 -> Magnitude-Angle to Complex1/2
  Demux/2 -> Add4/2, Magnitude-Angle to Complex2/2
  Add4/1 -> Magnitude-Angle to Complex3/2
  Demux/3 -> Magnitude-Angle to Complex4/2, Add5/2
  Add5/1 -> Magnitude-Angle to Complex5/2
  [VL25] -> Gain4/1
  Memory1/1 -> Complex to Magnitude-Angle/1
  Product/1 -> Gain2/1, Magnitude-Angle to Complex4/1, Magnitude-Angle to Complex2/1
  Product1/1 -> Magnitude-Angle to Complex1/1, Magnitude-Angle to Complex5/1, Magnitude-Angle to Complex3/1
  Gain4/1 -> Memory1/1
  Gain2/1 -> Magnitude-Angle to Complex/1
  Demux1/2 -> To Workspace3/1
  [VL25] -> Memory2/1
  Demux1/1 -> To Workspace1/1
  Demux2/2 -> To Workspace5/1
  Memory2/1 -> Power (Phasor)2/1
  i_current3/1 -> Mux1/1
  Demux2/3 -> To Workspace6/1
  Demux1/3 -> To Workspace4/1
  Power (Phasor)2/2 -> Demux2/1
  Demux2/1 -> To Workspace2/1
  i_current1/1 -> Mux1/2
  i_current2/1 -> Mux1/3
  Power (Phasor)2/1 -> Demux1/1
  Mux1/1 -> Power (Phasor)2/2
  connections:
  Three-Phase V-I Measurement2/RConn1 -- Controlled Current Source/RConn1 -- Three-Phase Series RLC Branch2/LConn1
  Three-Phase V-I Measurement2/RConn2 -- Controlled Current Source1/RConn1 -- Three-Phase Series RLC Branch2/LConn2
  Three-Phase V-I Measurement2/RConn3 -- Controlled Current Source2/RConn1 -- Three-Phase Series RLC Branch2/LConn3
  Controlled Current Source1/LConn1 -- Three-Phase Series RLC Branch2/RConn3 -- Three-Phase Series RLC Branch2/RConn1 -- Controlled Current Source/LConn1 -- Three-Phase Series RLC Branch2/RConn2 -- Ground2/LConn1 -- Controlled Current Source2/LConn1
  c+/RConn1 -- i_current2/RConn1
  Three-Phase V-I Measurement2/LConn1 -- i_current3/LConn1
  Three-Phase V-I Measurement2/LConn3 -- i_current2/LConn1
  a+/RConn1 -- i_current3/RConn1
  b+/RConn1 -- i_current1/RConn1
  Three-Phase V-I Measurement2/LConn2 -- i_current1/LConn1

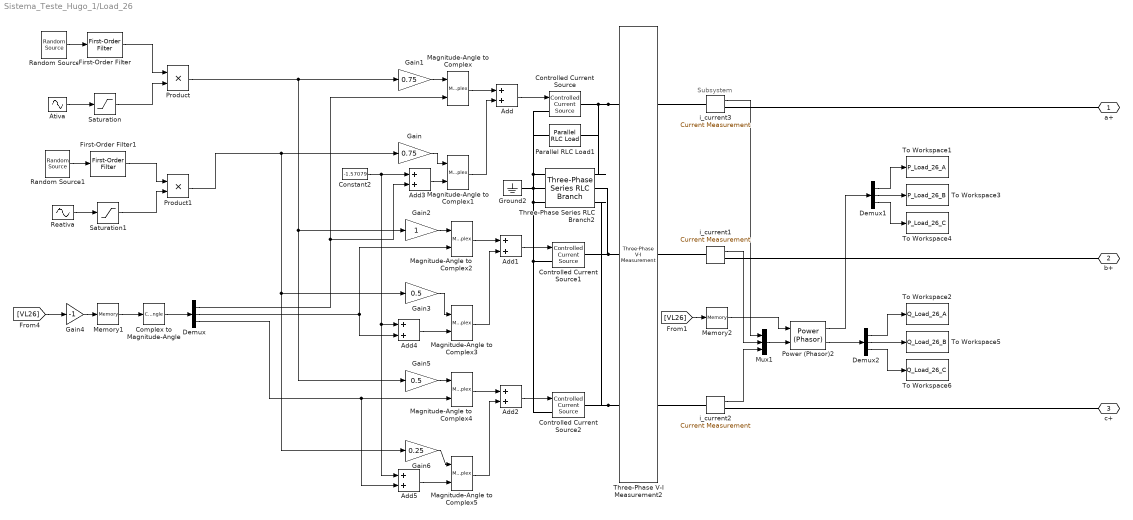
== system Sistema_Teste_Hugo_1/Load_26 ==
  note: Subsystem
  Add{,1..5} (6 alike) : Sum
  Ativa : Sin  Amplitude=11  Frequency=6.9e-5  Phase=-3.14  SampleTime=0
  Complex to Magnitude-Angle : ComplexToMagnitudeAngle  Output=Angle
  Constant2 : Constant  Value=-1.57079
  Controlled Current Source : powerlib/Electrical Sources/Controlled Current Source  Initialize=off  Source_Type=AC  Amplitude=0  Phase=0  Frequency=0  Measurements=None
      settings: SourceProductName=Simscape Electrical
  Controlled Current Source1 : powerlib/Electrical Sources/Controlled Current Source  Initialize=off  Source_Type=AC  Amplitude=0  Phase=0  Frequency=0  Measurements=None
      settings: SourceProductName=Simscape Electrical
  Controlled Current Source2 : powerlib/Electrical Sources/Controlled Current Source  Initialize=off  Source_Type=AC  Amplitude=0  Phase=0  Frequency=0  Measurements=None
      settings: SourceProductName=Simscape Electrical
  Demux : Demux  Outputs=3
  Demux1 : Demux  Outputs=3
  Demux2 : Demux  Outputs=3
  First-Order Filter : powerlib_meascontrol/Filters/First-Order Filter  FilterType=Lowpass  Tc=200  Ts=0  Initialize=on  Vac_Init=[0, 0, 60]  Vdc_Init=1  PlotResponse=off  FreqRange="[0,  200,  1]"
      settings: SourceProductName=Simscape Electrical
  First-Order Filter1 : powerlib_meascontrol/Filters/First-Order Filter  FilterType=Lowpass  Tc=400  Ts=0  Initialize=on  Vac_Init=[0, 0, 60]  Vdc_Init=1  PlotResponse=off  FreqRange="[0,  200,  1]"
      settings: SourceProductName=Simscape Electrical
  Gain : Gain  Gain=0.75
  Gain1 : Gain  Gain=0.75
  Gain2 : Gain
  Gain3 : Gain  Gain=0.5
  Gain4 : Gain  Gain=-1
  Gain5 : Gain  Gain=0.5
  Gain6 : Gain  Gain=0.25
  Ground2 : powerlib/Elements/Ground  LConnTagsString=a
      settings: SourceProductName=Simscape Electrical
  Magnitude-Angle to Complex{,1..5} (6 alike) : MagnitudeAngleToComplex
  Memory1 : Memory
  Memory2 : Memory
  Mux1 : Mux  Inputs=3
  Parallel RLC Load1 : powerlib/Elements/Parallel RLC Load  LConnTagsString=a  RConnTagsString=__new0  NominalVoltage=127  NominalFrequency=60  ActivePower=100  InductivePower=40  CapacitivePower=0  Setx0=off  InitialVoltage=0  SetiL0=off  InitialCurrent=0  Measurements=None  LoadType=constant Z
      settings: AttributesFormatString=\n  SourceProductName=Simscape Electrical  SourceProductBaseCode=PS
  Power (Phasor)2 : powerlib_meascontrol/Measurements/Power (Phasor)
      settings: SourceProductName=Simscape Electrical  SourceProductBaseCode=PS
  Product : Product
  Product1 : Product
  Random Source : dspsrcs4/Random Source  SrcType=Uniform  NormMethod=Ziggurat  CltLength=12  MinVal=0.6  MaxVal=1  MeanVal=0  VarVal=1  RepMode=Repeatable  rawSeed=1  IsInherit=off  SampMode=Discrete  SampTime=200  SampFrame=1  DataType=Single  OutComplex=Real  OutputFrames=on
  Random Source1 : dspsrcs4/Random Source  SrcType=Uniform  NormMethod=Ziggurat  CltLength=12  MinVal=0.7  MaxVal=1.05  MeanVal=0  VarVal=1  RepMode=Repeatable  rawSeed=1  IsInherit=off  SampMode=Discrete  SampTime=400  SampFrame=1  DataType=Single  OutComplex=Real  OutputFrames=on
  Reativa : Sin  Amplitude=5  Frequency=6.9e-5  Phase=-3.14  SampleTime=0
  Saturation : Saturate  UpperLimit=36  LowerLimit=5.5
  Saturation1 : Saturate  UpperLimit=10  LowerLimit=4
  Three-Phase Series RLC Branch2 : powerlib/Elements/Three-Phase Series RLC Branch  LConnTagsString=A|B|C  RConnTagsString=A|B|C  BranchType=RC  Resistance=0.0001  Inductance=5.46e-6  Capacitance=1e-9  Measurements=None
      settings: SourceProductName=Simscape Electrical
  Three-Phase V-I Measurement2 : powerlib/Measurements/Three-Phase V-I Measurement  VoltageMeasurement=phase-to-ground  SetLabelV=on  LabelV=VL26  Vpu=off  VpuLL=off  CurrentMeasurement=no  SetLabelI=on  LabelI=IL26  Ipu=off  Pbase=100e6  Vbase=500e3  OutputType=Complex  PhasorSimulation=on  PSBequivalent=0
      settings: SourceProductName=Simscape Electrical
  To Workspace1 : ToWorkspace  VariableName=P_Load_26_A  SampleTime=-1
  To Workspace2 : ToWorkspace  VariableName=Q_Load_26_A  SampleTime=-1
  To Workspace3 : ToWorkspace  VariableName=P_Load_26_B  SampleTime=-1
  To Workspace4 : ToWorkspace  VariableName=P_Load_26_C  SampleTime=-1
  To Workspace5 : ToWorkspace  VariableName=Q_Load_26_B  SampleTime=-1
  To Workspace6 : ToWorkspace  VariableName=Q_Load_26_C  SampleTime=-1
  i_current1 : powerlib/Measurements/Current Measurement  PhasorSimulation=on  OutputType=Complex  PSBequivalent=0
      settings: SourceProductName=Simscape Electrical
  i_current2 : powerlib/Measurements/Current Measurement  PhasorSimulation=on  OutputType=Complex  PSBequivalent=0
      settings: SourceProductName=Simscape Electrical
  i_current3 : powerlib/Measurements/Current Measurement  PhasorSimulation=on  OutputType=Complex  PSBequivalent=0
      settings: SourceProductName=Simscape Electrical
  a+ : PMIOPort  Side=Right
  b+ : PMIOPort  Port=2  Side=Right
  c+ : PMIOPort  Port=3  Side=Right
  wires:
  Ativa/1 -> Saturation/1
  Saturation/1 -> Product/2
  Random Source/1 -> First-Order Filter/1
  First-Order Filter/1 -> Product/1
  Reativa/1 -> Saturation1/1
  First-Order Filter1/1 -> Product1/1
  Random Source1/1 -> First-Order Filter1/1
  Saturation1/1 -> Product1/2
  Add/1 -> Controlled Current Source/1
  Magnitude-Angle to Complex/1 -> Add/1
  Magnitude-Angle to Complex1/1 -> Add/2
  Add1/1 -> Controlled Current Source1/1
  Magnitude-Angle to Complex2/1 -> Add1/1
  Magnitude-Angle to Complex3/1 -> Add1/2
  Add2/1 -> Controlled Current Source2/1
  Magnitude-Angle to Complex4/1 -> Add2/1
  Magnitude-Angle to Complex5/1 -> Add2/2
  Complex to Magnitude-Angle/1 -> Demux/1
  Demux/1 -> Magnitude-Angle to Complex/2, Add3/2
  Constant2/1 -> Add5/1, Add4/1, Add3/1
  Add3/1 -> Magnitude-Angle to Complex1/2
  Demux/2 -> Add4/2, Magnitude-Angle to Complex2/2
  Add4/1 -> Magnitude-Angle to Complex3/2
  Demux/3 -> Magnitude-Angle to Complex4/2, Add5/2
  Add5/1 -> Magnitude-Angle to Complex5/2
  [VL26] -> Gain4/1
  Memory1/1 -> Complex to Magnitude-Angle/1
  Product/1 -> Gain1/1, Gain5/1, Gain2/1
  Product1/1 -> Gain6/1, Gain3/1, Gain/1
  Gain2/1 -> Magnitude-Angle to Complex2/1
  Gain3/1 -> Magnitude-Angle to Complex3/1
  Gain1/1 -> Magnitude-Angle to Complex/1
  Gain/1 -> Magnitude-Angle to Complex1/1
  Gain4/1 -> Memory1/1
  Gain5/1 -> Magnitude-Angle to Complex4/1
  Gain6/1 -> Magnitude-Angle to Complex5/1
  [VL26] -> Memory2/1
  Demux2/2 -> To Workspace5/1
  Memory2/1 -> Power (Phasor)2/1
  Demux1/1 -> To Workspace1/1
  i_current2/1 -> Mux1/3
  i_current1/1 -> Mux1/2
  Power (Phasor)2/1 -> Demux1/1
  Demux1/2 -> To Workspace3/1
  i_current3/1 -> Mux1/1
  Mux1/1 -> Power (Phasor)2/2
  Power (Phasor)2/2 -> Demux2/1
  Demux1/3 -> To Workspace4/1
  Demux2/1 -> To Workspace2/1
  Demux2/3 -> To Workspace6/1
  connections:
  Three-Phase V-I Measurement2/RConn1 -- Controlled Current Source/RConn1 -- Parallel RLC Load1/LConn1 -- Three-Phase Series RLC Branch2/LConn1
  Three-Phase V-I Measurement2/RConn2 -- Controlled Current Source1/RConn1 -- Three-Phase Series RLC Branch2/LConn2
  Three-Phase V-I Measurement2/RConn3 -- Controlled Current Source2/RConn1 -- Three-Phase Series RLC Branch2/LConn3
  Controlled Current Source1/LConn1 -- Controlled Current Source2/LConn1 -- Three-Phase Series RLC Branch2/RConn3 -- Three-Phase Series RLC Branch2/RConn2 -- Ground2/LConn1 -- Three-Phase Series RLC Branch2/RConn1 -- Controlled Current Source/LConn1 -- Parallel RLC Load1/RConn1
  Three-Phase V-I Measurement2/LConn3 -- i_current2/LConn1
  b+/RConn1 -- i_current1/RConn1
  Three-Phase V-I Measurement2/LConn2 -- i_current1/LConn1
  Three-Phase V-I Measurement2/LConn1 -- i_current3/LConn1
  c+/RConn1 -- i_current2/RConn1
  a+/RConn1 -- i_current3/RConn1
